simulink library "Word_Multiplexers_Lib"  (R2023a)
settings: Solver=ode45  StartTime=0.0  StopTime=10.0  RelTol=1e-3  EnableMultiTasking=on
settings Model: Creator=uzivatel  LastModifiedBy=Jozko Mrkvicka
settings SolverCC: AlgebraicLoopSolver=TrustRegion
settings DataIOCC: LimitDataPoints=on  SaveFormat=Array  ReturnWorkspaceOutputs=off
settings OptimizationCC: LifeSpan=inf
settings DebuggingCC: UnderspecifiedInitializationDetection=Classic  MergeDetectMultiDrivingBlocksExec=none  SolverPrmCheckMsg=warning  UnconnectedInputMsg=warning  UnconnectedOutputMsg=warning  UnconnectedLineMsg=warning  StateNameClashWarn=warning  SFUnexpectedBacktrackingDiag=warning  SFNoUnconditionalDefaultTransitionDiag=warning  ArithmeticOperatorsInVariantConditions=warning
settings HardwareCC: ProdBitPerPointer=32  ProdBitPerSizeT=32  ProdBitPerPtrDiffT=32  ProdLargestAtomicFloat=None  ProdIntDivRoundTo=Undefined  ProdEndianess=Unspecified  ProdWordSize=32  ProdHWDeviceType=32-bit Generic
settings ModelReferenceCC: EnableRefExpFcnMdlSchedulingChecks=on  PropagateSignalLabelsOutOfModel=off
settings SFSimCC: SimUseLocalCustomCode=off  CustomCodeUndefinedFunction=UseInterfaceOnly
settings RTWCC: RTWUseLocalCustomCode=off
settings CodeAppCC: StateflowObjectComments=on
settings GRTTargetCC: TargetLangStandard=C89/C90 (ANSI)
settings ConfigComp: CovMetricSettings=dw  CovSaveCumulativeToWorkspaceVar=on  CovSaveSingleToWorkspaceVar=on  CovExternalEMLEnable=off

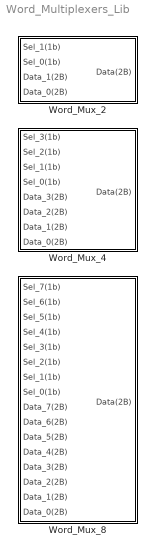
== system Word_Multiplexers_Lib ==
  Word_Mux_2 : Subsystem
  Word_Mux_4 : Subsystem
  Word_Mux_8 : Subsystem

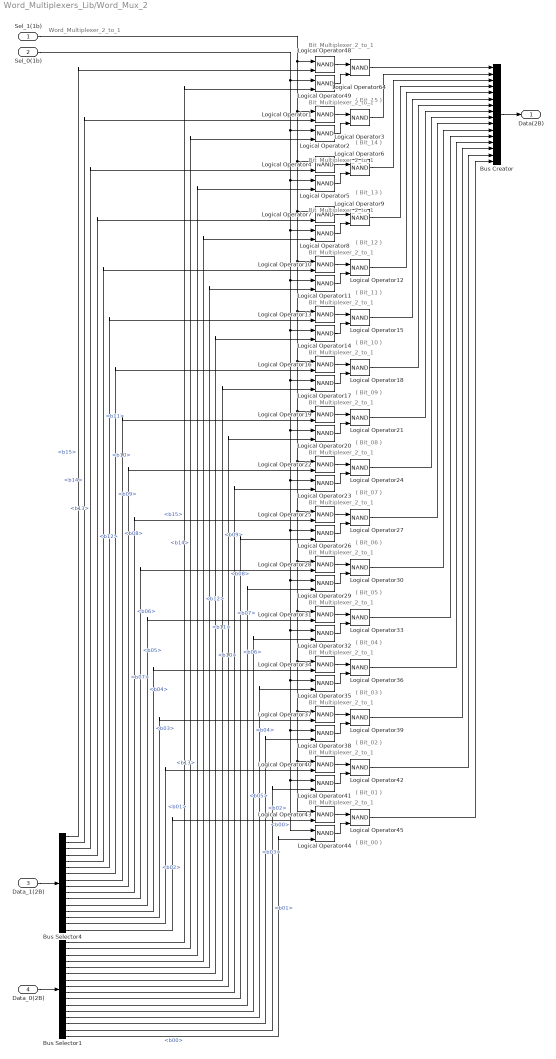
== system Word_Multiplexers_Lib/Word_Mux_2 ==
  note: ( Bit_15 )
  note: Bit_Multiplexer_2_to_1
  note: Bit_Multiplexer_2_to_1
  note: ( Bit_14 )
  note: Bit_Multiplexer_2_to_1
  note: ( Bit_13 )
  note: Bit_Multiplexer_2_to_1
  note: ( Bit_12 )
  note: Bit_Multiplexer_2_to_1
  note: ( Bit_11 )
  note: Bit_Multiplexer_2_to_1
  note: ( Bit_10 )
  note: Bit_Multiplexer_2_to_1
  note: ( Bit_09 )
  note: Bit_Multiplexer_2_to_1
  note: ( Bit_08 )
  note: Bit_Multiplexer_2_to_1
  note: ( Bit_07 )
  note: Bit_Multiplexer_2_to_1
  note: ( Bit_06 )
  note: Bit_Multiplexer_2_to_1
  note: ( Bit_05 )
  note: Bit_Multiplexer_2_to_1
  note: ( Bit_04 )
  note: Bit_Multiplexer_2_to_1
  note: ( Bit_03 )
  note: Bit_Multiplexer_2_to_1
  note: ( Bit_02 )
  note: Bit_Multiplexer_2_to_1
  note: ( Bit_01 )
  note: Bit_Multiplexer_2_to_1
  note: ( Bit_00 )
  note: Word_Multiplexer_2_to_1
  Sel_1(1b) : Inport
  Sel_0(1b) : Inport  Port=2
  Data_1(2B) : Inport  Port=3
  Data_0(2B) : Inport  Port=4
  Bus Creator : BusCreator  Inputs=16
  Bus Selector1 : BusSelector  OutputSignals=b15,b14,b13,b12,b11,b10,b09,b08,b07,b06,b05,b04,b03,b02,b01,b00
  Bus Selector4 : BusSelector  OutputSignals=b15,b14,b13,b12,b11,b10,b09,b08,b07,b06,b05,b04,b03,b02,b01,b00
  Logical Operator{1..2,4..5,7..8,10..11,13..14,16..17,19..20,22..23,25..26,28..29,31..32,34..35,37..38,40..41,43..44,48..49} (32 alike) : Logic  Operator=NAND  IconShape=distinctive  AllPortsSameDT=off  OutDataTypeStr=boolean
  Logical Operator{3,6,9,12,15,18,21,24,27,30,33,36,39,42,45,64} (16 alike) : Logic  Operator=NAND  IconShape=distinctive  OutDataTypeStr=boolean
  Data(2B) : Outport
  wires:
  Data_1(2B)/1 -> Bus Selector4/1
  Data_0(2B)/1 -> Bus Selector1/1
  Bus Creator/1 -> Data(2B)/1
  Bus Selector1/16 -> Logical Operator44/2  "<b00>"
  Bus Selector4/16 -> Logical Operator43/2  "<b00>"
  Bus Selector1/15 -> Logical Operator41/2  "<b01>"
  Bus Selector4/15 -> Logical Operator40/2  "<b01>"
  Bus Selector1/14 -> Logical Operator38/2  "<b02>"
  Bus Selector4/14 -> Logical Operator37/2  "<b02>"
  Bus Selector1/13 -> Logical Operator35/2  "<b03>"
  Bus Selector4/13 -> Logical Operator34/2  "<b03>"
  Bus Selector1/12 -> Logical Operator32/2  "<b04>"
  Bus Selector4/12 -> Logical Operator31/2  "<b04>"
  Bus Selector1/11 -> Logical Operator29/2  "<b05>"
  Bus Selector4/11 -> Logical Operator28/2  "<b05>"
  Bus Selector1/10 -> Logical Operator26/2  "<b06>"
  Bus Selector4/10 -> Logical Operator25/2  "<b06>"
  Bus Selector1/9 -> Logical Operator23/2  "<b07>"
  Bus Selector4/9 -> Logical Operator22/2  "<b07>"
  Bus Selector1/8 -> Logical Operator20/2  "<b08>"
  Bus Selector4/8 -> Logical Operator19/2  "<b08>"
  Bus Selector1/7 -> Logical Operator17/2  "<b09>"
  Bus Selector4/7 -> Logical Operator16/2  "<b09>"
  Bus Selector1/6 -> Logical Operator14/2  "<b10>"
  Bus Selector4/6 -> Logical Operator13/2  "<b10>"
  Bus Selector1/5 -> Logical Operator11/2  "<b11>"
  Bus Selector4/5 -> Logical Operator10/2  "<b11>"
  Bus Selector1/4 -> Logical Operator8/2  "<b12>"
  Bus Selector4/4 -> Logical Operator7/2  "<b12>"
  Bus Selector1/3 -> Logical Operator5/2  "<b13>"
  Bus Selector4/3 -> Logical Operator4/2  "<b13>"
  Bus Selector1/2 -> Logical Operator2/2  "<b14>"
  Bus Selector4/2 -> Logical Operator1/2  "<b14>"
  Bus Selector1/1 -> Logical Operator49/2  "<b15>"
  Bus Selector4/1 -> Logical Operator48/2  "<b15>"
  Logical Operator64/1 -> Bus Creator/1
  Sel_0(1b)/1 -> Logical Operator44/1, Logical Operator41/1, Logical Operator38/1, Logical Operator35/1, Logical Operator32/1, Logical Operator29/1, Logical Operator26/1, Logical Operator23/1, Logical Operator20/1, Logical Operator17/1, Logical Operator14/1, Logical Operator11/1, Logical Operator8/1, Logical Operator5/1, Logical Operator2/1, Logical Operator49/1
  Sel_1(1b)/1 -> Logical Operator37/1, Logical Operator40/1, Logical Operator43/1, Logical Operator34/1, Logical Operator31/1, Logical Operator28/1, Logical Operator25/1, Logical Operator22/1, Logical Operator19/1, Logical Operator16/1, Logical Operator13/1, Logical Operator10/1, Logical Operator7/1, Logical Operator4/1, Logical Operator1/1, Logical Operator48/1
  Logical Operator3/1 -> Bus Creator/2
  Logical Operator6/1 -> Bus Creator/3
  Logical Operator9/1 -> Bus Creator/4
  Logical Operator12/1 -> Bus Creator/5
  Logical Operator15/1 -> Bus Creator/6
  Logical Operator18/1 -> Bus Creator/7
  Logical Operator21/1 -> Bus Creator/8
  Logical Operator24/1 -> Bus Creator/9
  Logical Operator27/1 -> Bus Creator/10
  Logical Operator30/1 -> Bus Creator/11
  Logical Operator33/1 -> Bus Creator/12
  Logical Operator36/1 -> Bus Creator/13
  Logical Operator39/1 -> Bus Creator/14
  Logical Operator42/1 -> Bus Creator/15
  Logical Operator45/1 -> Bus Creator/16
  Logical Operator48/1 -> Logical Operator64/1
  Logical Operator49/1 -> Logical Operator64/2
  Logical Operator2/1 -> Logical Operator3/2
  Logical Operator1/1 -> Logical Operator3/1
  Logical Operator5/1 -> Logical Operator6/2
  Logical Operator4/1 -> Logical Operator6/1
  Logical Operator8/1 -> Logical Operator9/2
  Logical Operator7/1 -> Logical Operator9/1
  Logical Operator11/1 -> Logical Operator12/2
  Logical Operator10/1 -> Logical Operator12/1
  Logical Operator14/1 -> Logical Operator15/2
  Logical Operator13/1 -> Logical Operator15/1
  Logical Operator17/1 -> Logical Operator18/2
  Logical Operator16/1 -> Logical Operator18/1
  Logical Operator20/1 -> Logical Operator21/2
  Logical Operator19/1 -> Logical Operator21/1
  Logical Operator23/1 -> Logical Operator24/2
  Logical Operator22/1 -> Logical Operator24/1
  Logical Operator26/1 -> Logical Operator27/2
  Logical Operator25/1 -> Logical Operator27/1
  Logical Operator29/1 -> Logical Operator30/2
  Logical Operator28/1 -> Logical Operator30/1
  Logical Operator32/1 -> Logical Operator33/2
  Logical Operator31/1 -> Logical Operator33/1
  Logical Operator35/1 -> Logical Operator36/2
  Logical Operator34/1 -> Logical Operator36/1
  Logical Operator38/1 -> Logical Operator39/2
  Logical Operator37/1 -> Logical Operator39/1
  Logical Operator41/1 -> Logical Operator42/2
  Logical Operator40/1 -> Logical Operator42/1
  Logical Operator44/1 -> Logical Operator45/2
  Logical Operator43/1 -> Logical Operator45/1

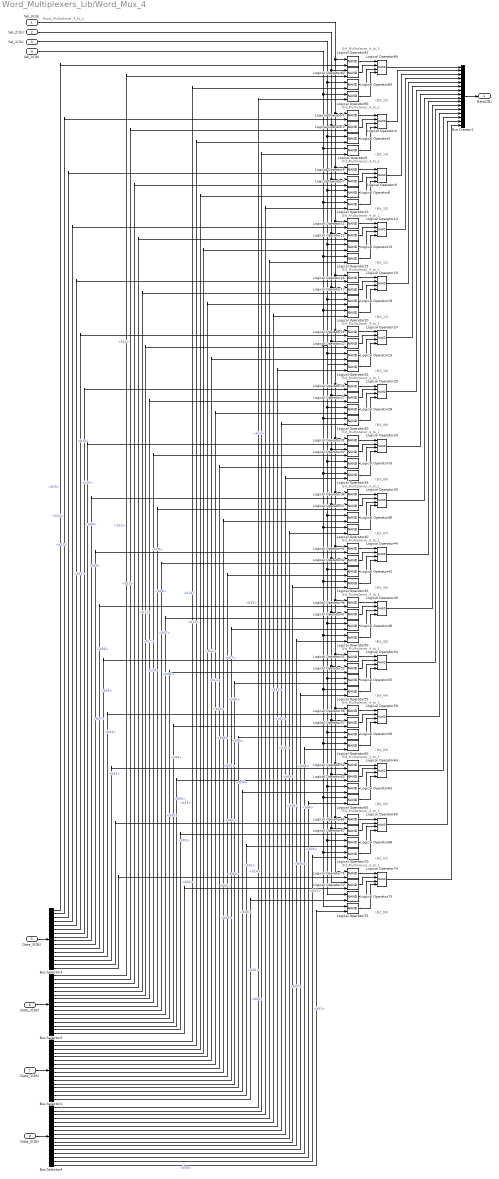
== system Word_Multiplexers_Lib/Word_Mux_4 ==
  note: Bit_Multiplexer_4_to_1
  note: (Bit_15)
  note: (Bit_14)
  note: Bit_Multiplexer_4_to_1
  note: (Bit_13)
  note: Bit_Multiplexer_4_to_1
  note: (Bit_12)
  note: Bit_Multiplexer_4_to_1
  note: (Bit_11)
  note: Bit_Multiplexer_4_to_1
  note: (Bit_10)
  note: Bit_Multiplexer_4_to_1
  note: (Bit_09)
  note: Bit_Multiplexer_4_to_1
  note: (Bit_08)
  note: Bit_Multiplexer_4_to_1
  note: (Bit_07)
  note: Bit_Multiplexer_4_to_1
  note: (Bit_06)
  note: Bit_Multiplexer_4_to_1
  note: (Bit_05)
  note: Bit_Multiplexer_4_to_1
  note: (Bit_04)
  note: Bit_Multiplexer_4_to_1
  note: (Bit_03)
  note: Bit_Multiplexer_4_to_1
  note: (Bit_02)
  note: Bit_Multiplexer_4_to_1
  note: (Bit_01)
  note: Bit_Multiplexer_4_to_1
  note: (Bit_00)
  note: Bit_Multiplexer_4_to_1
  note: Word_Multiplexer_4_to_1
  Sel_3(1b) : Inport
  Sel_2(1b) : Inport  Port=2
  Sel_1(1b) : Inport  Port=3
  Sel_0(1b) : Inport  Port=4
  Data_3(2B) : Inport  Port=5
  Data_2(2B) : Inport  Port=6
  Data_1(2B) : Inport  Port=7
  Data_0(2B) : Inport  Port=8
  Bus Creator1 : BusCreator  Inputs=16
  Bus Selector{1..4} (4 alike) : BusSelector  OutputSignals=b15,b14,b13,b12,b11,b10,b09,b08,b07,b06,b05,b04,b03,b02,b01,b00
  Logical Operator{1..3,5..8,10..13,15..18,20..23,25..28,30..33,35..38,40..43,45..48,50..53,55..58,60..63,65..68,70..73,75,81..83,85} (64 alike) : Logic  Operator=NAND  IconShape=distinctive  AllPortsSameDT=off  OutDataTypeStr=boolean
  Logical Operator{4,9,14,19,24,29,34,39,44,49,54,59,64,69,74,84} (16 alike) : Logic  Operator=NAND  Inputs=4  IconShape=distinctive  OutDataTypeStr=boolean
  Data(2B) : Outport
  wires:
  Data_3(2B)/1 -> Bus Selector3/1
  Data_2(2B)/1 -> Bus Selector2/1
  Data_1(2B)/1 -> Bus Selector1/1
  Data_0(2B)/1 -> Bus Selector4/1
  Bus Creator1/1 -> Data(2B)/1
  Bus Selector4/16 -> Logical Operator75/2  "<b00>"
  Bus Selector1/16 -> Logical Operator73/2  "<b00>"
  Bus Selector2/16 -> Logical Operator72/2  "<b00>"
  Bus Selector3/16 -> Logical Operator71/2  "<b00>"
  Bus Selector4/15 -> Logical Operator70/2  "<b01>"
  Bus Selector1/15 -> Logical Operator68/2  "<b01>"
  Bus Selector2/15 -> Logical Operator67/2  "<b01>"
  Bus Selector3/15 -> Logical Operator66/2  "<b01>"
  Bus Selector4/14 -> Logical Operator65/2  "<b02>"
  Bus Selector1/14 -> Logical Operator63/2  "<b02>"
  Bus Selector2/14 -> Logical Operator62/2  "<b02>"
  Bus Selector3/14 -> Logical Operator61/2  "<b02>"
  Bus Selector4/13 -> Logical Operator60/2  "<b03>"
  Bus Selector1/13 -> Logical Operator58/2  "<b03>"
  Bus Selector2/13 -> Logical Operator57/2  "<b03>"
  Bus Selector3/13 -> Logical Operator56/2  "<b03>"
  Bus Selector4/12 -> Logical Operator55/2  "<b04>"
  Bus Selector1/12 -> Logical Operator53/2  "<b04>"
  Bus Selector2/12 -> Logical Operator52/2  "<b04>"
  Bus Selector3/12 -> Logical Operator51/2  "<b04>"
  Bus Selector4/11 -> Logical Operator50/2  "<b05>"
  Bus Selector1/11 -> Logical Operator48/2  "<b05>"
  Bus Selector2/11 -> Logical Operator47/2  "<b05>"
  Bus Selector3/11 -> Logical Operator46/2  "<b05>"
  Bus Selector4/10 -> Logical Operator45/2  "<b06>"
  Bus Selector1/10 -> Logical Operator43/2  "<b06>"
  Bus Selector2/10 -> Logical Operator42/2  "<b06>"
  Bus Selector3/10 -> Logical Operator41/2  "<b06>"
  Bus Selector4/9 -> Logical Operator40/2  "<b07>"
  Bus Selector1/9 -> Logical Operator38/2  "<b07>"
  Bus Selector2/9 -> Logical Operator37/2  "<b07>"
  Bus Selector3/9 -> Logical Operator36/2  "<b07>"
  Bus Selector4/8 -> Logical Operator35/2  "<b08>"
  Bus Selector1/8 -> Logical Operator33/2  "<b08>"
  Bus Selector2/8 -> Logical Operator32/2  "<b08>"
  Bus Selector3/8 -> Logical Operator31/2  "<b08>"
  Bus Selector4/7 -> Logical Operator30/2  "<b09>"
  Bus Selector1/7 -> Logical Operator28/2  "<b09>"
  Bus Selector2/7 -> Logical Operator27/2  "<b09>"
  Bus Selector3/7 -> Logical Operator26/2  "<b09>"
  Bus Selector4/6 -> Logical Operator25/2  "<b10>"
  Bus Selector1/6 -> Logical Operator23/2  "<b10>"
  Bus Selector2/6 -> Logical Operator22/2  "<b10>"
  Bus Selector3/6 -> Logical Operator21/2  "<b10>"
  Bus Selector4/5 -> Logical Operator20/2  "<b11>"
  Bus Selector1/5 -> Logical Operator18/2  "<b11>"
  Bus Selector2/5 -> Logical Operator17/2  "<b11>"
  Bus Selector3/5 -> Logical Operator16/2  "<b11>"
  Bus Selector4/4 -> Logical Operator15/2  "<b12>"
  Bus Selector1/4 -> Logical Operator13/2  "<b12>"
  Bus Selector2/4 -> Logical Operator12/2  "<b12>"
  Bus Selector3/4 -> Logical Operator11/2  "<b12>"
  Bus Selector4/3 -> Logical Operator10/2  "<b13>"
  Bus Selector1/3 -> Logical Operator8/2  "<b13>"
  Bus Selector2/3 -> Logical Operator7/2  "<b13>"
  Bus Selector3/3 -> Logical Operator6/2  "<b13>"
  Bus Selector4/2 -> Logical Operator5/2  "<b14>"
  Bus Selector1/2 -> Logical Operator3/2  "<b14>"
  Bus Selector2/2 -> Logical Operator2/2  "<b14>"
  Bus Selector3/2 -> Logical Operator1/2  "<b14>"
  Bus Selector4/1 -> Logical Operator85/2  "<b15>"
  Bus Selector1/1 -> Logical Operator83/2  "<b15>"
  Bus Selector2/1 -> Logical Operator82/2  "<b15>"
  Bus Selector3/1 -> Logical Operator81/2  "<b15>"
  Sel_3(1b)/1 -> Logical Operator71/1, Logical Operator66/1, Logical Operator61/1, Logical Operator56/1, Logical Operator51/1, Logical Operator46/1, Logical Operator41/1, Logical Operator36/1, Logical Operator31/1, Logical Operator26/1, Logical Operator21/1, Logical Operator16/1, Logical Operator11/1, Logical Operator6/1, Logical Operator1/1, Logical Operator81/1
  Sel_2(1b)/1 -> Logical Operator82/1, Logical Operator2/1, Logical Operator72/1, Logical Operator67/1, Logical Operator62/1, Logical Operator57/1, Logical Operator52/1, Logical Operator47/1, Logical Operator42/1, Logical Operator37/1, Logical Operator32/1, Logical Operator27/1, Logical Operator22/1, Logical Operator17/1, Logical Operator12/1, Logical Operator7/1
  Sel_0(1b)/1 -> Logical Operator75/1, Logical Operator70/1, Logical Operator65/1, Logical Operator60/1, Logical Operator55/1, Logical Operator50/1, Logical Operator45/1, Logical Operator40/1, Logical Operator35/1, Logical Operator30/1, Logical Operator25/1, Logical Operator20/1, Logical Operator15/1, Logical Operator10/1, Logical Operator5/1, Logical Operator85/1
  Sel_1(1b)/1 -> Logical Operator73/1, Logical Operator68/1, Logical Operator63/1, Logical Operator58/1, Logical Operator53/1, Logical Operator48/1, Logical Operator43/1, Logical Operator38/1, Logical Operator33/1, Logical Operator28/1, Logical Operator23/1, Logical Operator18/1, Logical Operator13/1, Logical Operator8/1, Logical Operator3/1, Logical Operator83/1
  Logical Operator81/1 -> Logical Operator84/1
  Logical Operator83/1 -> Logical Operator84/3
  Logical Operator82/1 -> Logical Operator84/2
  Logical Operator85/1 -> Logical Operator84/4
  Logical Operator3/1 -> Logical Operator4/3
  Logical Operator5/1 -> Logical Operator4/4
  Logical Operator1/1 -> Logical Operator4/1
  Logical Operator2/1 -> Logical Operator4/2
  Logical Operator8/1 -> Logical Operator9/3
  Logical Operator10/1 -> Logical Operator9/4
  Logical Operator6/1 -> Logical Operator9/1
  Logical Operator7/1 -> Logical Operator9/2
  Logical Operator13/1 -> Logical Operator14/3
  Logical Operator15/1 -> Logical Operator14/4
  Logical Operator11/1 -> Logical Operator14/1
  Logical Operator12/1 -> Logical Operator14/2
  Logical Operator18/1 -> Logical Operator19/3
  Logical Operator20/1 -> Logical Operator19/4
  Logical Operator16/1 -> Logical Operator19/1
  Logical Operator17/1 -> Logical Operator19/2
  Logical Operator23/1 -> Logical Operator24/3
  Logical Operator25/1 -> Logical Operator24/4
  Logical Operator21/1 -> Logical Operator24/1
  Logical Operator22/1 -> Logical Operator24/2
  Logical Operator28/1 -> Logical Operator29/3
  Logical Operator30/1 -> Logical Operator29/4
  Logical Operator26/1 -> Logical Operator29/1
  Logical Operator27/1 -> Logical Operator29/2
  Logical Operator33/1 -> Logical Operator34/3
  Logical Operator35/1 -> Logical Operator34/4
  Logical Operator31/1 -> Logical Operator34/1
  Logical Operator32/1 -> Logical Operator34/2
  Logical Operator38/1 -> Logical Operator39/3
  Logical Operator40/1 -> Logical Operator39/4
  Logical Operator36/1 -> Logical Operator39/1
  Logical Operator37/1 -> Logical Operator39/2
  Logical Operator43/1 -> Logical Operator44/3
  Logical Operator45/1 -> Logical Operator44/4
  Logical Operator41/1 -> Logical Operator44/1
  Logical Operator42/1 -> Logical Operator44/2
  Logical Operator48/1 -> Logical Operator49/3
  Logical Operator50/1 -> Logical Operator49/4
  Logical Operator46/1 -> Logical Operator49/1
  Logical Operator47/1 -> Logical Operator49/2
  Logical Operator53/1 -> Logical Operator54/3
  Logical Operator55/1 -> Logical Operator54/4
  Logical Operator51/1 -> Logical Operator54/1
  Logical Operator52/1 -> Logical Operator54/2
  Logical Operator58/1 -> Logical Operator59/3
  Logical Operator60/1 -> Logical Operator59/4
  Logical Operator56/1 -> Logical Operator59/1
  Logical Operator57/1 -> Logical Operator59/2
  Logical Operator63/1 -> Logical Operator64/3
  Logical Operator65/1 -> Logical Operator64/4
  Logical Operator61/1 -> Logical Operator64/1
  Logical Operator62/1 -> Logical Operator64/2
  Logical Operator68/1 -> Logical Operator69/3
  Logical Operator70/1 -> Logical Operator69/4
  Logical Operator66/1 -> Logical Operator69/1
  Logical Operator67/1 -> Logical Operator69/2
  Logical Operator73/1 -> Logical Operator74/3
  Logical Operator75/1 -> Logical Operator74/4
  Logical Operator71/1 -> Logical Operator74/1
  Logical Operator72/1 -> Logical Operator74/2
  Logical Operator84/1 -> Bus Creator1/1
  Logical Operator4/1 -> Bus Creator1/2
  Logical Operator9/1 -> Bus Creator1/3
  Logical Operator14/1 -> Bus Creator1/4
  Logical Operator19/1 -> Bus Creator1/5
  Logical Operator24/1 -> Bus Creator1/6
  Logical Operator29/1 -> Bus Creator1/7
  Logical Operator34/1 -> Bus Creator1/8
  Logical Operator39/1 -> Bus Creator1/9
  Logical Operator44/1 -> Bus Creator1/10
  Logical Operator49/1 -> Bus Creator1/11
  Logical Operator54/1 -> Bus Creator1/12
  Logical Operator59/1 -> Bus Creator1/13
  Logical Operator64/1 -> Bus Creator1/14
  Logical Operator69/1 -> Bus Creator1/15
  Logical Operator74/1 -> Bus Creator1/16

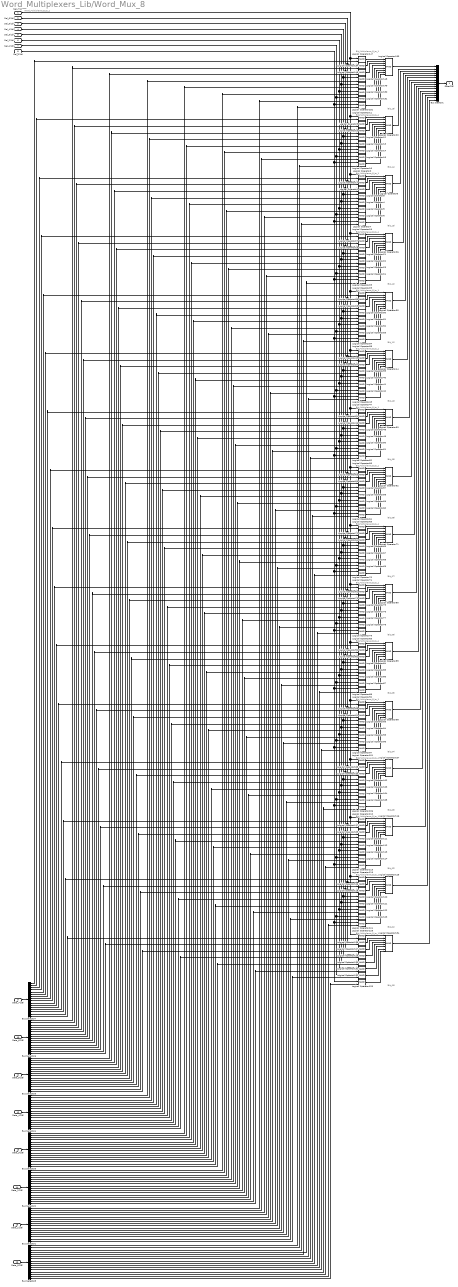
== system Word_Multiplexers_Lib/Word_Mux_8 ==
  note: Bit_Multiplexer_8_to_1
  note: (Bit_15)
  note: Bit_Multiplexer_8_to_1
  note: (Bit_14)
  note: Bit_Multiplexer_8_to_1
  note: (Bit_13)
  note: Bit_Multiplexer_8_to_1
  note: (Bit_12)
  note: Bit_Multiplexer_8_to_1
  note: (Bit_11)
  note: Bit_Multiplexer_8_to_1
  note: (Bit_10)
  note: Bit_Multiplexer_8_to_1
  note: (Bit_09)
  note: Bit_Multiplexer_8_to_1
  note: (Bit_08)
  note: Bit_Multiplexer_8_to_1
  note: (Bit_07)
  note: Bit_Multiplexer_8_to_1
  note: (Bit_06)
  note: Bit_Multiplexer_8_to_1
  note: (Bit_05)
  note: Bit_Multiplexer_8_to_1
  note: (Bit_04)
  note: Bit_Multiplexer_8_to_1
  note: (Bit_03)
  note: Bit_Multiplexer_8_to_1
  note: (Bit_02)
  note: Bit_Multiplexer_8_to_1
  note: (Bit_01)
  note: Bit_Multiplexer_8_to_1
  note: (Bit_00)
  note: Word_Multiplexer_8_to_1
  Sel_7(1b) : Inport
  Sel_6(1b) : Inport  Port=2
  Sel_5(1b) : Inport  Port=3
  Sel_4(1b) : Inport  Port=4
  Sel_3(1b) : Inport  Port=5
  Sel_2(1b) : Inport  Port=6
  Sel_1(1b) : Inport  Port=7
  Sel_0(1b) : Inport  Port=8
  Data_7(2B) : Inport  Port=9
  Data_6(2B) : Inport  Port=10
  Data_5(2B) : Inport  Port=11
  Data_4(2B) : Inport  Port=12
  Data_3(2B) : Inport  Port=13
  Data_2(2B) : Inport  Port=14
  Data_1(2B) : Inport  Port=15
  Data_0(2B) : Inport  Port=16
  Bus Creator1 : BusCreator  Inputs=16
  Bus Selector{1..8} (8 alike) : BusSelector  OutputSignals=b15,b14,b13,b12,b11,b10,b09,b08,b07,b06,b05,b04,b03,b02,b01,b00
  Logical Operator{1..7,9..19,21..25,27..34,36..43,45..52,54..61,63..70,72..79,81..88,90..97,99..106,108..115,117..124,126..133,135,146..152,154} (128 alike) : Logic  Operator=NAND  IconShape=distinctive  AllPortsSameDT=off  OutDataTypeStr=boolean
  Logical Operator{8,20,26,35,44,53,62,71,80,89,98,107,116,125,134,153} (16 alike) : Logic  Operator=NAND  Inputs=8  IconShape=distinctive  OutDataTypeStr=boolean
  Data(2B) : Outport
  wires:
  Bus Selector8/16 -> Logical Operator133/2  "<b00>"
  Bus Selector1/16 -> Logical Operator132/2  "<b00>"
  Bus Selector2/16 -> Logical Operator131/2  "<b00>"
  Bus Selector3/16 -> Logical Operator130/2  "<b00>"
  Bus Selector4/16 -> Logical Operator129/2  "<b00>"
  Bus Selector5/16 -> Logical Operator127/2  "<b00>"
  Bus Selector6/16 -> Logical Operator135/2  "<b00>"
  Bus Selector7/16 -> Logical Operator128/2  "<b00>"
  Bus Selector8/15 -> Logical Operator124/2  "<b01>"
  Bus Selector1/15 -> Logical Operator123/2  "<b01>"
  Bus Selector2/15 -> Logical Operator122/2  "<b01>"
  Bus Selector3/15 -> Logical Operator121/2  "<b01>"
  Bus Selector4/15 -> Logical Operator120/2  "<b01>"
  Bus Selector5/15 -> Logical Operator118/2  "<b01>"
  Bus Selector6/15 -> Logical Operator126/2  "<b01>"
  Bus Selector7/15 -> Logical Operator119/2  "<b01>"
  Bus Selector8/14 -> Logical Operator115/2  "<b02>"
  Bus Selector1/14 -> Logical Operator114/2  "<b02>"
  Bus Selector2/14 -> Logical Operator113/2  "<b02>"
  Bus Selector3/14 -> Logical Operator112/2  "<b02>"
  Bus Selector4/14 -> Logical Operator111/2  "<b02>"
  Bus Selector5/14 -> Logical Operator109/2  "<b02>"
  Bus Selector6/14 -> Logical Operator117/2  "<b02>"
  Bus Selector7/14 -> Logical Operator110/2  "<b02>"
  Bus Selector8/13 -> Logical Operator106/2  "<b03>"
  Bus Selector1/13 -> Logical Operator105/2  "<b03>"
  Bus Selector2/13 -> Logical Operator104/2  "<b03>"
  Bus Selector3/13 -> Logical Operator103/2  "<b03>"
  Bus Selector4/13 -> Logical Operator102/2  "<b03>"
  Bus Selector5/13 -> Logical Operator100/2  "<b03>"
  Bus Selector6/13 -> Logical Operator108/2  "<b03>"
  Bus Selector7/13 -> Logical Operator101/2  "<b03>"
  Bus Selector8/12 -> Logical Operator97/2  "<b04>"
  Bus Selector1/12 -> Logical Operator96/2  "<b04>"
  Bus Selector2/12 -> Logical Operator95/2  "<b04>"
  Bus Selector3/12 -> Logical Operator94/2  "<b04>"
  Bus Selector4/12 -> Logical Operator93/2  "<b04>"
  Bus Selector5/12 -> Logical Operator91/2  "<b04>"
  Bus Selector6/12 -> Logical Operator99/2  "<b04>"
  Bus Selector7/12 -> Logical Operator92/2  "<b04>"
  Bus Selector8/11 -> Logical Operator88/2  "<b05>"
  Bus Selector1/11 -> Logical Operator87/2  "<b05>"
  Bus Selector2/11 -> Logical Operator86/2  "<b05>"
  Bus Selector3/11 -> Logical Operator85/2  "<b05>"
  Bus Selector4/11 -> Logical Operator84/2  "<b05>"
  Bus Selector5/11 -> Logical Operator82/2  "<b05>"
  Bus Selector6/11 -> Logical Operator90/2  "<b05>"
  Bus Selector7/11 -> Logical Operator83/2  "<b05>"
  Bus Selector8/10 -> Logical Operator79/2  "<b06>"
  Bus Selector1/10 -> Logical Operator78/2  "<b06>"
  Bus Selector2/10 -> Logical Operator77/2  "<b06>"
  Bus Selector3/10 -> Logical Operator76/2  "<b06>"
  Bus Selector4/10 -> Logical Operator75/2  "<b06>"
  Bus Selector5/10 -> Logical Operator73/2  "<b06>"
  Bus Selector6/10 -> Logical Operator81/2  "<b06>"
  Bus Selector7/10 -> Logical Operator74/2  "<b06>"
  Bus Selector8/9 -> Logical Operator70/2  "<b07>"
  Bus Selector1/9 -> Logical Operator69/2  "<b07>"
  Bus Selector2/9 -> Logical Operator68/2  "<b07>"
  Bus Selector3/9 -> Logical Operator67/2  "<b07>"
  Bus Selector4/9 -> Logical Operator66/2  "<b07>"
  Bus Selector5/9 -> Logical Operator64/2  "<b07>"
  Bus Selector6/9 -> Logical Operator72/2  "<b07>"
  Bus Selector7/9 -> Logical Operator65/2  "<b07>"
  Bus Selector8/8 -> Logical Operator61/2  "<b08>"
  Bus Selector1/8 -> Logical Operator60/2  "<b08>"
  Bus Selector2/8 -> Logical Operator59/2  "<b08>"
  Bus Selector3/8 -> Logical Operator58/2  "<b08>"
  Bus Selector4/8 -> Logical Operator57/2  "<b08>"
  Bus Selector5/8 -> Logical Operator55/2  "<b08>"
  Bus Selector6/8 -> Logical Operator63/2  "<b08>"
  Bus Selector7/8 -> Logical Operator56/2  "<b08>"
  Bus Selector8/7 -> Logical Operator52/2  "<b09>"
  Bus Selector1/7 -> Logical Operator51/2  "<b09>"
  Bus Selector2/7 -> Logical Operator50/2  "<b09>"
  Bus Selector3/7 -> Logical Operator49/2  "<b09>"
  Bus Selector4/7 -> Logical Operator48/2  "<b09>"
  Bus Selector5/7 -> Logical Operator46/2  "<b09>"
  Bus Selector6/7 -> Logical Operator54/2  "<b09>"
  Bus Selector7/7 -> Logical Operator47/2  "<b09>"
  Bus Selector8/6 -> Logical Operator43/2  "<b10>"
  Bus Selector1/6 -> Logical Operator42/2  "<b10>"
  Bus Selector2/6 -> Logical Operator41/2  "<b10>"
  Bus Selector3/6 -> Logical Operator40/2  "<b10>"
  Bus Selector4/6 -> Logical Operator39/2  "<b10>"
  Bus Selector5/6 -> Logical Operator37/2  "<b10>"
  Bus Selector6/6 -> Logical Operator45/2  "<b10>"
  Bus Selector7/6 -> Logical Operator38/2  "<b10>"
  Bus Selector8/5 -> Logical Operator34/2  "<b11>"
  Bus Selector1/5 -> Logical Operator33/2  "<b11>"
  Bus Selector2/5 -> Logical Operator32/2  "<b11>"
  Bus Selector3/5 -> Logical Operator31/2  "<b11>"
  Bus Selector4/5 -> Logical Operator30/2  "<b11>"
  Bus Selector5/5 -> Logical Operator28/2  "<b11>"
  Bus Selector6/5 -> Logical Operator36/2  "<b11>"
  Bus Selector7/5 -> Logical Operator29/2  "<b11>"
  Bus Selector8/4 -> Logical Operator25/2  "<b12>"
  Bus Selector1/4 -> Logical Operator24/2  "<b12>"
  Bus Selector2/4 -> Logical Operator23/2  "<b12>"
  Bus Selector3/4 -> Logical Operator22/2  "<b12>"
  Bus Selector4/4 -> Logical Operator21/2  "<b12>"
  Bus Selector5/4 -> Logical Operator18/2  "<b12>"
  Bus Selector6/4 -> Logical Operator27/2  "<b12>"
  Bus Selector7/4 -> Logical Operator19/2  "<b12>"
  Bus Selector8/3 -> Logical Operator7/2  "<b13>"
  Bus Selector1/3 -> Logical Operator6/2  "<b13>"
  Bus Selector2/3 -> Logical Operator5/2  "<b13>"
  Bus Selector3/3 -> Logical Operator4/2  "<b13>"
  Bus Selector4/3 -> Logical Operator3/2  "<b13>"
  Bus Selector5/3 -> Logical Operator1/2  "<b13>"
  Bus Selector6/3 -> Logical Operator17/2  "<b13>"
  Bus Selector7/3 -> Logical Operator2/2  "<b13>"
  Bus Selector8/2 -> Logical Operator16/2  "<b14>"
  Bus Selector1/2 -> Logical Operator15/2  "<b14>"
  Bus Selector2/2 -> Logical Operator14/2  "<b14>"
  Bus Selector3/2 -> Logical Operator13/2  "<b14>"
  Bus Selector4/2 -> Logical Operator12/2  "<b14>"
  Bus Selector5/2 -> Logical Operator10/2  "<b14>"
  Bus Selector6/2 -> Logical Operator9/2  "<b14>"
  Bus Selector7/2 -> Logical Operator11/2  "<b14>"
  Bus Selector8/1 -> Logical Operator152/2  "<b15>"
  Bus Selector1/1 -> Logical Operator151/2  "<b15>"
  Bus Selector2/1 -> Logical Operator150/2  "<b15>"
  Bus Selector3/1 -> Logical Operator149/2  "<b15>"
  Bus Selector4/1 -> Logical Operator148/2  "<b15>"
  Bus Selector5/1 -> Logical Operator146/2  "<b15>"
  Bus Selector6/1 -> Logical Operator154/2  "<b15>"
  Bus Selector7/1 -> Logical Operator147/2  "<b15>"
  Sel_7(1b)/1 -> Logical Operator147/1, Logical Operator11/1, Logical Operator128/1, Logical Operator119/1, Logical Operator110/1, Logical Operator101/1, Logical Operator92/1, Logical Operator83/1, Logical Operator74/1, Logical Operator65/1, Logical Operator56/1, Logical Operator47/1, Logical Operator38/1, Logical Operator29/1, Logical Operator19/1, Logical Operator2/1
  Sel_6(1b)/1 -> Logical Operator135/1, Logical Operator126/1, Logical Operator117/1, Logical Operator108/1, Logical Operator99/1, Logical Operator90/1, Logical Operator81/1, Logical Operator72/1, Logical Operator63/1, Logical Operator54/1, Logical Operator45/1, Logical Operator36/1, Logical Operator27/1, Logical Operator17/1, Logical Operator9/1, Logical Operator154/1
  Sel_4(1b)/1 -> Logical Operator129/1, Logical Operator120/1, Logical Operator111/1, Logical Operator102/1, Logical Operator93/1, Logical Operator84/1, Logical Operator75/1, Logical Operator66/1, Logical Operator57/1, Logical Operator48/1, Logical Operator39/1, Logical Operator30/1, Logical Operator21/1, Logical Operator3/1, Logical Operator12/1, Logical Operator148/1
  Sel_3(1b)/1 -> Logical Operator76/1, Logical Operator85/1, Logical Operator112/1, Logical Operator121/1, Logical Operator130/1, Logical Operator103/1, Logical Operator94/1, Logical Operator67/1, Logical Operator58/1, Logical Operator49/1, Logical Operator40/1, Logical Operator31/1, Logical Operator22/1, Logical Operator4/1, Logical Operator13/1, Logical Operator149/1
  Sel_2(1b)/1 -> Logical Operator32/1, Logical Operator41/1, Logical Operator131/1, Logical Operator122/1, Logical Operator113/1, Logical Operator104/1, Logical Operator95/1, Logical Operator86/1, Logical Operator77/1, Logical Operator68/1, Logical Operator59/1, Logical Operator50/1, Logical Operator23/1, Logical Operator5/1, Logical Operator14/1, Logical Operator150/1
  Sel_0(1b)/1 -> Logical Operator133/1, Logical Operator124/1, Logical Operator115/1, Logical Operator106/1, Logical Operator97/1, Logical Operator88/1, Logical Operator79/1, Logical Operator70/1, Logical Operator61/1, Logical Operator52/1, Logical Operator43/1, Logical Operator34/1, Logical Operator25/1, Logical Operator7/1, Logical Operator16/1, Logical Operator152/1
  Sel_1(1b)/1 -> Logical Operator132/1, Logical Operator123/1, Logical Operator114/1, Logical Operator105/1, Logical Operator96/1, Logical Operator87/1, Logical Operator78/1, Logical Operator69/1, Logical Operator60/1, Logical Operator51/1, Logical Operator42/1, Logical Operator33/1, Logical Operator24/1, Logical Operator6/1, Logical Operator15/1, Logical Operator151/1
  Sel_5(1b)/1 -> Logical Operator109/1, Logical Operator118/1, Logical Operator127/1, Logical Operator100/1, Logical Operator91/1, Logical Operator82/1, Logical Operator73/1, Logical Operator64/1, Logical Operator55/1, Logical Operator46/1, Logical Operator37/1, Logical Operator28/1, Logical Operator18/1, Logical Operator1/1, Logical Operator10/1, Logical Operator146/1
  Logical Operator148/1 -> Logical Operator153/4
  Logical Operator149/1 -> Logical Operator153/5
  Logical Operator150/1 -> Logical Operator153/6
  Logical Operator152/1 -> Logical Operator153/8
  Logical Operator154/1 -> Logical Operator153/2
  Logical Operator151/1 -> Logical Operator153/7
  Logical Operator146/1 -> Logical Operator153/3
  Logical Operator147/1 -> Logical Operator153/1
  Logical Operator12/1 -> Logical Operator20/4
  Logical Operator13/1 -> Logical Operator20/5
  Logical Operator14/1 -> Logical Operator20/6
  Logical Operator16/1 -> Logical Operator20/8
  Logical Operator9/1 -> Logical Operator20/2
  Logical Operator15/1 -> Logical Operator20/7
  Logical Operator10/1 -> Logical Operator20/3
  Logical Operator11/1 -> Logical Operator20/1
  Logical Operator3/1 -> Logical Operator8/4
  Logical Operator4/1 -> Logical Operator8/5
  Logical Operator5/1 -> Logical Operator8/6
  Logical Operator7/1 -> Logical Operator8/8
  Logical Operator17/1 -> Logical Operator8/2
  Logical Operator6/1 -> Logical Operator8/7
  Logical Operator1/1 -> Logical Operator8/3
  Logical Operator2/1 -> Logical Operator8/1
  Logical Operator21/1 -> Logical Operator26/4
  Logical Operator22/1 -> Logical Operator26/5
  Logical Operator23/1 -> Logical Operator26/6
  Logical Operator25/1 -> Logical Operator26/8
  Logical Operator27/1 -> Logical Operator26/2
  Logical Operator24/1 -> Logical Operator26/7
  Logical Operator18/1 -> Logical Operator26/3
  Logical Operator19/1 -> Logical Operator26/1
  Logical Operator30/1 -> Logical Operator35/4
  Logical Operator31/1 -> Logical Operator35/5
  Logical Operator32/1 -> Logical Operator35/6
  Logical Operator34/1 -> Logical Operator35/8
  Logical Operator36/1 -> Logical Operator35/2
  Logical Operator33/1 -> Logical Operator35/7
  Logical Operator28/1 -> Logical Operator35/3
  Logical Operator29/1 -> Logical Operator35/1
  Logical Operator39/1 -> Logical Operator44/4
  Logical Operator40/1 -> Logical Operator44/5
  Logical Operator41/1 -> Logical Operator44/6
  Logical Operator43/1 -> Logical Operator44/8
  Logical Operator45/1 -> Logical Operator44/2
  Logical Operator42/1 -> Logical Operator44/7
  Logical Operator37/1 -> Logical Operator44/3
  Logical Operator38/1 -> Logical Operator44/1
  Logical Operator48/1 -> Logical Operator53/4
  Logical Operator49/1 -> Logical Operator53/5
  Logical Operator50/1 -> Logical Operator53/6
  Logical Operator52/1 -> Logical Operator53/8
  Logical Operator54/1 -> Logical Operator53/2
  Logical Operator51/1 -> Logical Operator53/7
  Logical Operator46/1 -> Logical Operator53/3
  Logical Operator47/1 -> Logical Operator53/1
  Logical Operator57/1 -> Logical Operator62/4
  Logical Operator58/1 -> Logical Operator62/5
  Logical Operator59/1 -> Logical Operator62/6
  Logical Operator61/1 -> Logical Operator62/8
  Logical Operator63/1 -> Logical Operator62/2
  Logical Operator60/1 -> Logical Operator62/7
  Logical Operator55/1 -> Logical Operator62/3
  Logical Operator56/1 -> Logical Operator62/1
  Logical Operator66/1 -> Logical Operator71/4
  Logical Operator67/1 -> Logical Operator71/5
  Logical Operator68/1 -> Logical Operator71/6
  Logical Operator70/1 -> Logical Operator71/8
  Logical Operator72/1 -> Logical Operator71/2
  Logical Operator69/1 -> Logical Operator71/7
  Logical Operator64/1 -> Logical Operator71/3
  Logical Operator65/1 -> Logical Operator71/1
  Logical Operator75/1 -> Logical Operator80/4
  Logical Operator76/1 -> Logical Operator80/5
  Logical Operator77/1 -> Logical Operator80/6
  Logical Operator79/1 -> Logical Operator80/8
  Logical Operator81/1 -> Logical Operator80/2
  Logical Operator78/1 -> Logical Operator80/7
  Logical Operator73/1 -> Logical Operator80/3
  Logical Operator74/1 -> Logical Operator80/1
  Logical Operator84/1 -> Logical Operator89/4
  Logical Operator85/1 -> Logical Operator89/5
  Logical Operator86/1 -> Logical Operator89/6
  Logical Operator88/1 -> Logical Operator89/8
  Logical Operator90/1 -> Logical Operator89/2
  Logical Operator87/1 -> Logical Operator89/7
  Logical Operator82/1 -> Logical Operator89/3
  Logical Operator83/1 -> Logical Operator89/1
  Logical Operator93/1 -> Logical Operator98/4
  Logical Operator94/1 -> Logical Operator98/5
  Logical Operator95/1 -> Logical Operator98/6
  Logical Operator97/1 -> Logical Operator98/8
  Logical Operator99/1 -> Logical Operator98/2
  Logical Operator96/1 -> Logical Operator98/7
  Logical Operator91/1 -> Logical Operator98/3
  Logical Operator92/1 -> Logical Operator98/1
  Logical Operator102/1 -> Logical Operator107/4
  Logical Operator103/1 -> Logical Operator107/5
  Logical Operator104/1 -> Logical Operator107/6
  Logical Operator106/1 -> Logical Operator107/8
  Logical Operator108/1 -> Logical Operator107/2
  Logical Operator105/1 -> Logical Operator107/7
  Logical Operator100/1 -> Logical Operator107/3
  Logical Operator101/1 -> Logical Operator107/1
  Logical Operator111/1 -> Logical Operator116/4
  Logical Operator112/1 -> Logical Operator116/5
  Logical Operator113/1 -> Logical Operator116/6
  Logical Operator115/1 -> Logical Operator116/8
  Logical Operator117/1 -> Logical Operator116/2
  Logical Operator114/1 -> Logical Operator116/7
  Logical Operator109/1 -> Logical Operator116/3
  Logical Operator110/1 -> Logical Operator116/1
  Logical Operator120/1 -> Logical Operator125/4
  Logical Operator121/1 -> Logical Operator125/5
  Logical Operator122/1 -> Logical Operator125/6
  Logical Operator124/1 -> Logical Operator125/8
  Logical Operator126/1 -> Logical Operator125/2
  Logical Operator123/1 -> Logical Operator125/7
  Logical Operator118/1 -> Logical Operator125/3
  Logical Operator119/1 -> Logical Operator125/1
  Logical Operator129/1 -> Logical Operator134/4
  Logical Operator130/1 -> Logical Operator134/5
  Logical Operator131/1 -> Logical Operator134/6
  Logical Operator133/1 -> Logical Operator134/8
  Logical Operator135/1 -> Logical Operator134/2
  Logical Operator132/1 -> Logical Operator134/7
  Logical Operator127/1 -> Logical Operator134/3
  Logical Operator128/1 -> Logical Operator134/1
  Logical Operator153/1 -> Bus Creator1/1
  Logical Operator20/1 -> Bus Creator1/2
  Logical Operator8/1 -> Bus Creator1/3
  Logical Operator26/1 -> Bus Creator1/4
  Logical Operator35/1 -> Bus Creator1/5
  Logical Operator44/1 -> Bus Creator1/6
  Logical Operator53/1 -> Bus Creator1/7
  Logical Operator62/1 -> Bus Creator1/8
  Logical Operator71/1 -> Bus Creator1/9
  Logical Operator80/1 -> Bus Creator1/10
  Logical Operator98/1 -> Bus Creator1/12
  Logical Operator89/1 -> Bus Creator1/11
  Logical Operator107/1 -> Bus Creator1/13
  Logical Operator116/1 -> Bus Creator1/14
  Logical Operator125/1 -> Bus Creator1/15
  Logical Operator134/1 -> Bus Creator1/16
  Bus Creator1/1 -> Data(2B)/1
  Data_7(2B)/1 -> Bus Selector7/1
  Data_6(2B)/1 -> Bus Selector6/1
  Data_5(2B)/1 -> Bus Selector5/1
  Data_4(2B)/1 -> Bus Selector4/1
  Data_3(2B)/1 -> Bus Selector3/1
  Data_2(2B)/1 -> Bus Selector2/1
  Data_1(2B)/1 -> Bus Selector1/1
  Data_0(2B)/1 -> Bus Selector8/1
